simulink model "CombinedPIDFuzzModified"  (R2016a)
settings: Solver=VariableStepAuto  StartTime=0.0  StopTime=10.0  RelTol=1e-3
values from neighbouring files (symbols this model uses):
  Bm = 0.002953    [April2code.mat]    (also in April6code.mat)
  GCE = 0.900162058346    [April2code.mat]    (also in April6code.mat = 0.875095724066)
  GCU = 0.001    [April2code.mat]    (also in April6code.mat)
  GE = 10    [April2code.mat]    (also in April6code.mat)
  GU = 0.499909983794    [April2code.mat]    (also in April6code.mat = 0.799912490428)
  Jm = 0.02215    [April2code.mat]    (also in April6code.mat)
  Kb = 1.28    [April2code.mat]    (also in April6code.mat)
  Kt = 1.28    [April2code.mat]    (also in April6code.mat)
  La = 0.1215    [April2code.mat]    (also in April6code.mat)
  Ra = 11.2    [April2code.mat]    (also in April6code.mat)
undefined symbols (not defined in the file or in its folder): DiscIntNeverNeededParam
libraries: fuzblock x1
settings Model: Creator=Dheeraj Singh  LastModifiedBy=Dheeraj Singh

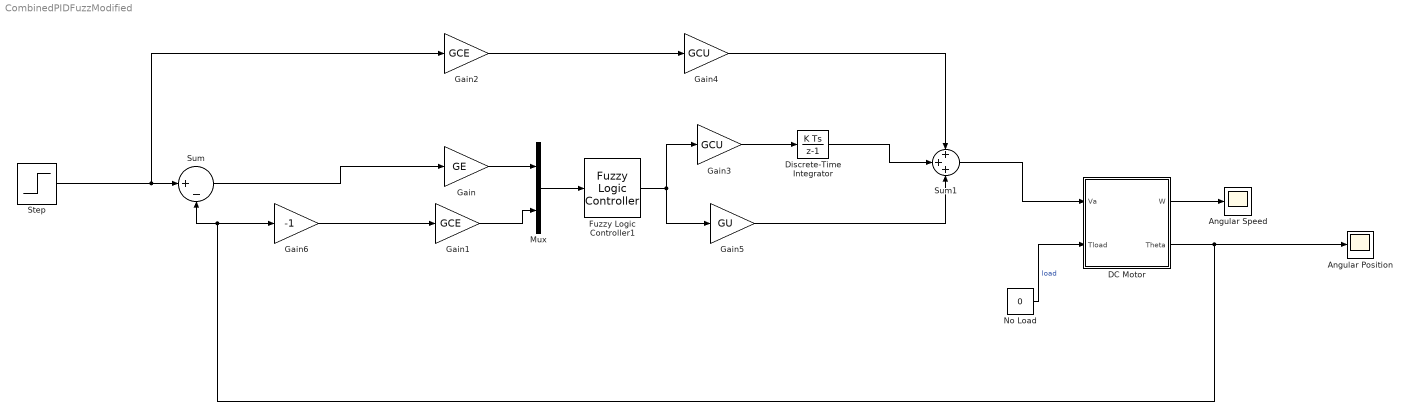
== system CombinedPIDFuzzModified ==
  Angular Position : Scope
  Angular Speed : Scope
  DC Motor : Subsystem
  Discrete-Time Integrator : DiscreteIntegrator  InitialConditionSetting=State (most efficient)  ICPrevOutput=DiscIntNeverNeededParam  ICPrevScaledInput=DiscIntNeverNeededParam
  Fuzzy Logic Controller1 : fuzblock/Fuzzy Logic  Controller  fis=Mam_centroid
  Gain : Gain  Gain=GE
  Gain1 : Gain  Gain=GCE
  Gain2 : Gain  Gain=GCE
  Gain3 : Gain  Gain=GCU
  Gain4 : Gain  Gain=GCU
  Gain5 : Gain  Gain=GU
  Gain6 : Gain  Gain=-1
  Mux : Mux  Inputs=2
  No Load : Constant  Value=0
  Step : Step  SampleTime=0
  Sum : Sum  Inputs=|+-
  Sum1 : Sum  Inputs=+++
  wires:
  No Load/1 -> DC Motor/2(Tload)  "load"
  DC Motor/1(W) -> Angular Speed/1
  Step/1 -> Sum/1, Gain2/1
  DC Motor/2(Theta) -> Sum/2, Gain6/1, Angular Position/1
  Gain/1 -> Mux/1
  Gain1/1 -> Mux/2
  Mux/1 -> Fuzzy Logic Controller1/1
  Gain2/1 -> Gain4/1
  Fuzzy Logic Controller1/1 -> Gain3/1, Gain5/1
  Gain3/1 -> Discrete-Time Integrator/1
  Sum/1 -> Gain/1
  Discrete-Time Integrator/1 -> Sum1/2
  Gain5/1 -> Sum1/3
  Gain4/1 -> Sum1/1
  Sum1/1 -> DC Motor/1(Va)
  Gain6/1 -> Gain1/1

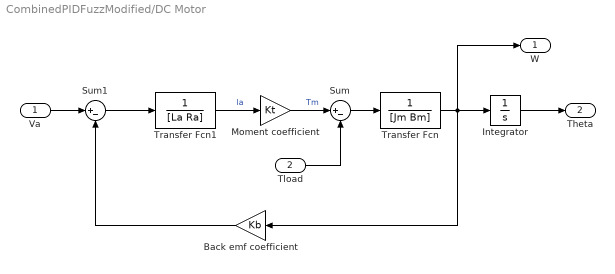
== system CombinedPIDFuzzModified/DC Motor ==
  Va : Inport
  Tload : Inport  Port=2
  Back emf coefficient : Gain  Gain=Kb
  Integrator : Integrator
  Moment coefficient : Gain  Gain=Kt
  Sum : Sum  Inputs=|+-
  Sum1 : Sum  Inputs=|+-
  Transfer Fcn : TransferFcn  Denominator=[Jm Bm]
  Transfer Fcn1 : TransferFcn  Denominator=[La Ra]
  W : Outport
  Theta : Outport  Port=2
  wires:
  Transfer Fcn1/1 -> Moment coefficient/1  "la"
  Sum/1 -> Transfer Fcn/1
  Va/1 -> Sum1/1
  Moment coefficient/1 -> Sum/1  "Tm"
  Transfer Fcn/1 -> W/1, Back emf coefficient/1, Integrator/1
  Integrator/1 -> Theta/1
  Tload/1 -> Sum/2
  Sum1/1 -> Transfer Fcn1/1
  Back emf coefficient/1 -> Sum1/2
